simulink model "sitlpmpc"  (R2025a)
settings: Solver=FixedStepAuto  StartTime=0.0  StopTime=inf  RelTol=1e-3  EnableMultiTasking=on
PreLoadFcn:
  | SampleTime = 1e-3;
  | isUsingSimulinkMixer=true;
libraries: px4Sensorslib x2, slpidlib x2, px4Peripheralslib x1
CloseFcn:
  | clear SampleTime;
settings Model: ExtModeTrigDuration=10  Creator=The MathWorks, Inc.  LastModifiedBy=aero
settings SolverCC: AlgebraicLoopSolver=TrustRegion  PositivePriorityOrder=on  MaxZcPerStep=1.0
settings OptimizationCC: EnhancedBackFolding=on  PassReuseOutputArgsAs=Individual arguments  ZeroExternalMemoryAtStartup=off  ZeroInternalMemoryAtStartup=off  MaxStackSize=64  OptimizeBlockOrder=speed  DifferentSizesBufferReuse=on  OptimizationCustomize=off  EfficientTunableParamExpr=on
settings DebuggingCC: ParameterPrecisionLossMsg=none  ParameterTunabilityLossMsg=error  UnconnectedInputMsg=warning  UnconnectedOutputMsg=warning  UnconnectedLineMsg=warning  SubsystemReferenceDiagnosticForUnitTest=warning
settings HardwareCC: ProdBitPerPointer=32.0  ProdBitPerSizeT=32.0  ProdBitPerPtrDiffT=32.0  ProdLargestAtomicInteger=Long  ProdLargestAtomicFloat=Double  ProdWordSize=32.0  ProdLongLongMode=on  ProdHWDeviceType=ARM Compatible->ARM Cortex
settings ModelReferenceCC: EnableRefExpFcnMdlSchedulingChecks=on
settings SFSimCC: MATLABDynamicMemAlloc=off  SimTargetLang=C++  SimDLTargetLibrary=mkl-dnn
settings RTWCC: SystemTargetFile=ert.tlc  HardwareBoard=PX4 Host Target  TLCOptions="-aInlineSetEventsForThisBaseRateFcn=TLC_FALSE -aSuppressMultiTaskScheduler=TLC_FALSE  -aRateBasedStepFcn=0"  TemplateMakefile=ert_default_tmf  Toolchain=GNU Tools for PX4 Autopilots  PortableWordSizes=on  TargetLang=C++  GPUComputeCapability=3.5  DLArmComputeVersion=19.05  Description=Embedded Coder
settings CodeAppCC: ForceParamTrailComments=on  IgnoreCustomStorageClasses=off  OperatorAnnotations=on  SimulinkDataObjDesc=on  SFDataObjDesc=on  InsertBlockDesc=on
settings ERTTargetCC: ExtModeTransport=2.0  InlinedParameterPlacement=Hierarchical

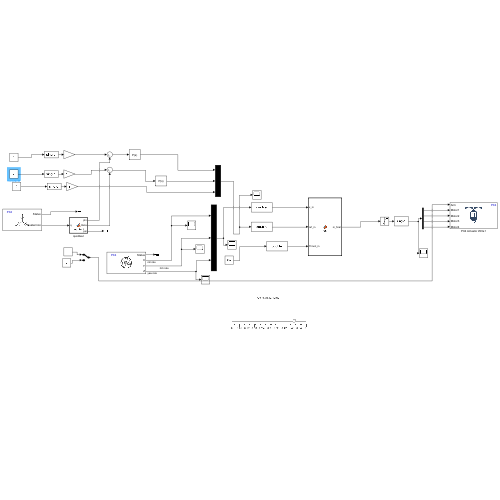
[thumbnail: Simulink's stored preview of the top-level diagram]
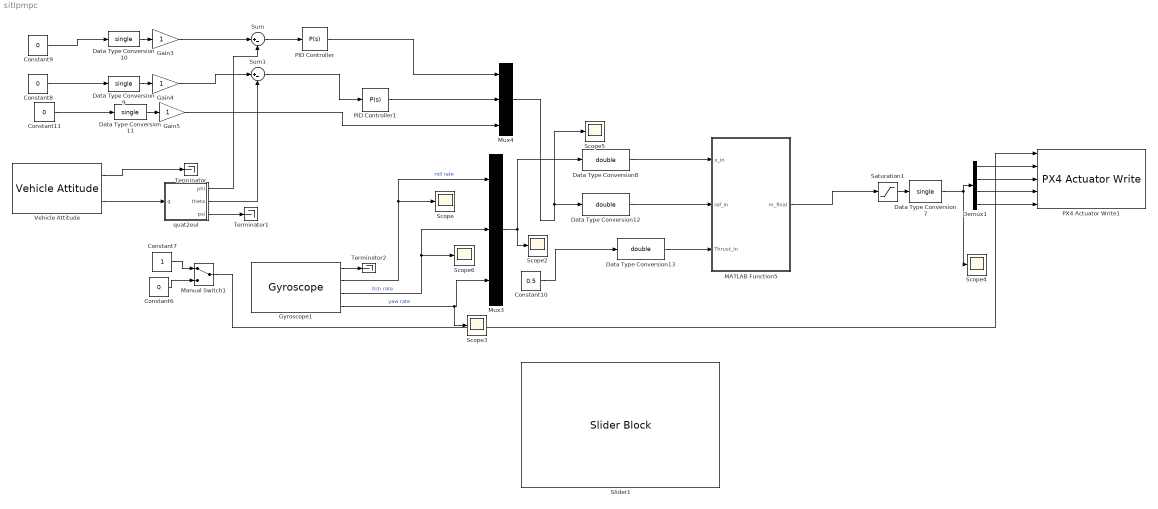
== system sitlpmpc ==
  Constant10 : Constant  Value=0.5
  Constant11 : Constant  Value=0
  Constant6 : Constant  Value=0  OutDataTypeStr=boolean
  Constant7 : Constant  OutDataTypeStr=boolean
  Constant8 : Constant  Value=0
  Constant9 : Constant  Value=0
  Data Type Conversion{7,9..11} (4 alike) : DataTypeConversion  OutDataTypeStr=single  SaturateOnIntegerOverflow=off  RndMeth=Floor
  Data Type Conversion12 : DataTypeConversion  OutDataTypeStr=double  SaturateOnIntegerOverflow=off  RndMeth=Floor  LockScale=on
  Data Type Conversion13 : DataTypeConversion  OutDataTypeStr=double  SaturateOnIntegerOverflow=off  RndMeth=Floor  LockScale=on
  Data Type Conversion8 : DataTypeConversion  OutDataTypeStr=double  SaturateOnIntegerOverflow=off  RndMeth=Floor  LockScale=on
  Demux1 : Demux
  Gain3 : Gain
  Gain4 : Gain
  Gain5 : Gain
  Gyroscope1 : px4Sensorslib/Gyroscope  uorbTimeStamp=off  BlockingMode=off  BlockTimeout=1e-3  sampleTime=0.001
  MATLAB Function5 : MATLAB Function  TreatAsAtomicUnit=on
  Manual Switch1 : ManualSwitch
  Mux3 : Mux  Inputs=3
  Mux4 : Mux  Inputs=3
  PID Controller : slpidlib/PID Controller  Controller=P  Form=Parallel  TimeDomain=Continuous-time  UseExternalTs=off  SampleTime=-1  IntegratorMethod=Forward Euler  FilterMethod=Forward Euler  ControllerParametersSource=internal  P=0.25  I=1  UseKiTs=off  D=0  UseExternalDerivativeSource=off  N=100  UseFilter=on  TunerSelectOption=Transfer Function Based (PID Tuner App)  InitialConditionSource=internal  InitialConditionForIntegrator=0  InitialConditionForFilter=0  DifferentiatorICPrevScaledInput=0  ExternalReset=none  TrackingMode=off  Kt=1  LimitOutput=off  SatLimitsSource=internal  UpperSaturationLimit=inf  LowerSaturationLimit=-inf  LinearizeAsGain=on  AntiWindupMode=none  Kb=1  LimitIntegrator=off  UpperIntegratorSaturationLimit=inf  LowerIntegratorSaturationLimit=-inf  POutMin=[]  POutMax=[]  IOutMin=[]  IOutMax=[]  DOutMin=[]  DOutMax=[]  NOutMin=[]  NOutMax=[]  SumOutMin=[]  SumOutMax=[]  SaturationOutMin=[]  SaturationOutMax=[]  PParamMin=[]  PParamMax=[]  IParamMin=[]  IParamMax=[]  DParamMin=[]  DParamMax=[]  NParamMin=[]  NParamMax=[]  KbParamMin=[]  KbParamMax=[]  KtParamMin=[]  KtParamMax=[]  KbOutMin=[]  KbOutMax=[]  KtOutMin=[]  KtOutMax=[]  IntegratorOutMin=[]  IntegratorOutMax=[]  FilterOutMin=[]  FilterOutMax=[]  SumI1OutMin=[]  SumI1OutMax=[]  SumI2OutMin=[]  SumI2OutMax=[]  SumI3OutMin=[]  SumI3OutMax=[]  SumI4OutMin=[]  SumI4OutMax=[]  SumDOutMin=[]  SumDOutMax=[]  DifferentiatorOutMin=[]  DifferentiatorOutMax=[]  FilterDiffOutCoefMin=[]  FilterDiffOutCoefMax=[]  ReciprocalOutMin=[]  ReciprocalOutMax=[]  SumDenOutMin=[]  SumDenOutMax=[]  SumNumOutMin=[]  SumNumOutMax=[]  DivideOutMin=[]  DivideOutMax=[]  UdiffTsProdOutMin=[]  UdiffTsProdOutMax=[]  NTsProdOutMin=[]  NTsProdOutMax=[]  UintegralTsProdOutMin=[]  UintegralTsProdOutMax=[]  UngainTsProdOutMin=[]  UngainTsProdOutMax=[]  ClampingZeroOutDataTypeStr=Inherit: Inherit via back propagation  ClampingZeroOutMin=[]  ClampingZeroOutMax=[]  FilterDenConstantOutDataTypeStr=Inherit: Inherit via back propagation  FilterDenConstantOutMin=[]  FilterDenConstantOutMax=[]  PCopyOutDataTypeStr=Inherit: Inherit via back propagation  PCopyOutMin=[]  PCopyOutMax=[]  NCopyOutDataTypeStr=Inherit: Inherit via back propagation  NCopyOutMin=[]  NCopyOutMax=[]  IntegratorContinuousStateAttributes=''  IntegratorStateMustResolveToSignalObject=off  IntegratorRTWStateStorageClass=Auto  FilterContinuousStateAttributes=''  FilterStateMustResolveToSignalObject=off  FilterRTWStateStorageClass=Auto  ParallelPVariant=InternalParameters  IdealPVariant=Disabled  IVariant=Disabled  DVariant=Disabled  IntegratorVariant=Disabled  SatVariant=Disabled  AWVariant=Disabled  PCopyVariant=Disabled  TRVariant=Disabled  FdbkBlocksVariant=Forward  IdealPFdbkVariant=Disabled  SatFdbkVariant=Disabled  DerivativeFilterVariant=Disabled  NVariant=Disabled  NCopyVariant=Disabled_SignalSpec  FilterICVariant=Disabled  IntegratorICVariant=Disabled  ExternalResetVariant=Disabled  TRSumVariant=Passthrough  SumFdbkVariant=Disabled  SumVariant=Passthrough_P  TsampFilterVariant=InternalTs  TsampNgainVariant=Passthrough  TsampIntegralVariant=Disabled_SignalSpec  ExternalSaturationOutDataTypeStr=Inherit: Same as second input  DerivativeSourceVariant=Disabled  PreIntVariant=InternalPreInt
  PID Controller1 : slpidlib/PID Controller  Controller=P  Form=Parallel  TimeDomain=Continuous-time  UseExternalTs=off  SampleTime=-1  IntegratorMethod=Forward Euler  FilterMethod=Forward Euler  ControllerParametersSource=internal  P=0.25  I=1  UseKiTs=off  D=0  UseExternalDerivativeSource=off  N=100  UseFilter=on  TunerSelectOption=Transfer Function Based (PID Tuner App)  InitialConditionSource=internal  InitialConditionForIntegrator=0  InitialConditionForFilter=0  DifferentiatorICPrevScaledInput=0  ExternalReset=none  TrackingMode=off  Kt=1  LimitOutput=off  SatLimitsSource=internal  UpperSaturationLimit=inf  LowerSaturationLimit=-inf  LinearizeAsGain=on  AntiWindupMode=none  Kb=1  LimitIntegrator=off  UpperIntegratorSaturationLimit=inf  LowerIntegratorSaturationLimit=-inf  POutMin=[]  POutMax=[]  IOutMin=[]  IOutMax=[]  DOutMin=[]  DOutMax=[]  NOutMin=[]  NOutMax=[]  SumOutMin=[]  SumOutMax=[]  SaturationOutMin=[]  SaturationOutMax=[]  PParamMin=[]  PParamMax=[]  IParamMin=[]  IParamMax=[]  DParamMin=[]  DParamMax=[]  NParamMin=[]  NParamMax=[]  KbParamMin=[]  KbParamMax=[]  KtParamMin=[]  KtParamMax=[]  KbOutMin=[]  KbOutMax=[]  KtOutMin=[]  KtOutMax=[]  IntegratorOutMin=[]  IntegratorOutMax=[]  FilterOutMin=[]  FilterOutMax=[]  SumI1OutMin=[]  SumI1OutMax=[]  SumI2OutMin=[]  SumI2OutMax=[]  SumI3OutMin=[]  SumI3OutMax=[]  SumI4OutMin=[]  SumI4OutMax=[]  SumDOutMin=[]  SumDOutMax=[]  DifferentiatorOutMin=[]  DifferentiatorOutMax=[]  FilterDiffOutCoefMin=[]  FilterDiffOutCoefMax=[]  ReciprocalOutMin=[]  ReciprocalOutMax=[]  SumDenOutMin=[]  SumDenOutMax=[]  SumNumOutMin=[]  SumNumOutMax=[]  DivideOutMin=[]  DivideOutMax=[]  UdiffTsProdOutMin=[]  UdiffTsProdOutMax=[]  NTsProdOutMin=[]  NTsProdOutMax=[]  UintegralTsProdOutMin=[]  UintegralTsProdOutMax=[]  UngainTsProdOutMin=[]  UngainTsProdOutMax=[]  ClampingZeroOutDataTypeStr=Inherit: Inherit via back propagation  ClampingZeroOutMin=[]  ClampingZeroOutMax=[]  FilterDenConstantOutDataTypeStr=Inherit: Inherit via back propagation  FilterDenConstantOutMin=[]  FilterDenConstantOutMax=[]  PCopyOutDataTypeStr=Inherit: Inherit via back propagation  PCopyOutMin=[]  PCopyOutMax=[]  NCopyOutDataTypeStr=Inherit: Inherit via back propagation  NCopyOutMin=[]  NCopyOutMax=[]  IntegratorContinuousStateAttributes=''  IntegratorStateMustResolveToSignalObject=off  IntegratorRTWStateStorageClass=Auto  FilterContinuousStateAttributes=''  FilterStateMustResolveToSignalObject=off  FilterRTWStateStorageClass=Auto  ParallelPVariant=InternalParameters  IdealPVariant=Disabled  IVariant=Disabled  DVariant=Disabled  IntegratorVariant=Disabled  SatVariant=Disabled  AWVariant=Disabled  PCopyVariant=Disabled  TRVariant=Disabled  FdbkBlocksVariant=Forward  IdealPFdbkVariant=Disabled  SatFdbkVariant=Disabled  DerivativeFilterVariant=Disabled  NVariant=Disabled  NCopyVariant=Disabled_SignalSpec  FilterICVariant=Disabled  IntegratorICVariant=Disabled  ExternalResetVariant=Disabled  TRSumVariant=Passthrough  SumFdbkVariant=Disabled  SumVariant=Passthrough_P  TsampFilterVariant=InternalTs  TsampNgainVariant=Passthrough  TsampIntegralVariant=Disabled_SignalSpec  ExternalSaturationOutDataTypeStr=Inherit: Same as second input  DerivativeSourceVariant=Disabled  PreIntVariant=InternalPreInt
  PX4 Actuator Write1 : px4Peripheralslib/PX4 Actuator Write  Motor1Enable=on  Motor2Enable=on  Motor3Enable=on  Motor4Enable=on  Motor5Enable=off  Motor6Enable=off  Motor7Enable=off  Motor8Enable=off  Motor9Enable=off  Motor10Enable=off  Motor11Enable=off  Motor12Enable=off  IsMotorArray=off  Servo1Enable=off  Servo2Enable=off  Servo3Enable=off  Servo4Enable=off  Servo5Enable=off  Servo6Enable=off  Servo7Enable=off  Servo8Enable=off  IsServoArray=off
  Saturation1 : Saturate  UpperLimit=1  LowerLimit=0
  Scope{,2..6} (6 alike) : Scope
      Scope settings: ActiveDisplayYMinimum=-0.048647073097527027  ActiveDisplayYMaximum=0.043675837107002735
      Scope2 settings: ActiveDisplayYMinimum=-0.62053689360618591  ActiveDisplayYMaximum=0.55083355307579041
      Scope3 settings: ActiveDisplayYMinimum=-1  ActiveDisplayYMaximum=1  DataLoggingVariableName=ScopeData3
      Scope4 settings: ActiveDisplayYMinimum=0.057510972242240666  ActiveDisplayYMaximum=0.55490137269269046  DataLoggingVariableName=ScopeData4
      Scope5 settings: ActiveDisplayYMinimum=-3.3246570702222038  ActiveDisplayYMaximum=4.6404233658291121  DataLoggingVariableName=ScopeData5
      Scope6 settings: ActiveDisplayYMinimum=-1  ActiveDisplayYMaximum=1  DataLoggingVariableName=ScopeData6
  Slider1 : SliderBlock  ScaleMax=0.6
  Sum : Sum  Inputs=|+-
  Sum1 : Sum  Inputs=|+-
  Terminator : Terminator
  Terminator1 : Terminator
  Terminator2 : Terminator
  Vehicle Attitude : px4Sensorslib/Vehicle Attitude  rollRate=off  pitchRate=off  yawRate=off  quaternion=on  uorbTimeStamp=off  BlockingMode=off  BlockTimeout=0.001  sampleTime=0.001
  quat2eul : MATLAB Function  TreatAsAtomicUnit=on
  wires:
  Data Type Conversion13/1 -> MATLAB Function5/3(Thrust_in)
  Data Type Conversion8/1 -> MATLAB Function5/1(x_in)
  Demux1/1 -> PX4 Actuator Write1/2
  Constant11/1 -> Data Type Conversion11/1
  Data Type Conversion10/1 -> Gain3/1
  Mux3/1 -> Scope2/1, Data Type Conversion8/1
  Constant8/1 -> Data Type Conversion9/1
  Data Type Conversion9/1 -> Gain4/1
  Constant9/1 -> Data Type Conversion10/1
  Constant10/1 -> Data Type Conversion13/1
  Mux4/1 -> Scope5/1, Data Type Conversion12/1
  Data Type Conversion7/1 -> Demux1/1, Scope4/1
  Demux1/4 -> PX4 Actuator Write1/5
  Saturation1/1 -> Data Type Conversion7/1
  Gyroscope1/4 -> Scope3/1, Mux3/3  "yaw rate"
  Gyroscope1/1 -> Terminator2/1
  Gyroscope1/2 -> Scope/1, Mux3/1  "roll rate"
  Constant6/1 -> Manual Switch1/2
  Data Type Conversion12/1 -> MATLAB Function5/2(ref_in)
  Constant7/1 -> Manual Switch1/1
  Demux1/3 -> PX4 Actuator Write1/4
  Data Type Conversion11/1 -> Gain5/1
  Gyroscope1/3 -> Mux3/2, Scope6/1  "itch rate"
  Demux1/2 -> PX4 Actuator Write1/3
  MATLAB Function5/1(m_final) -> Saturation1/1
  Manual Switch1/1 -> PX4 Actuator Write1/1
  Vehicle Attitude/2 -> quat2eul/1(q)
  Vehicle Attitude/1 -> Terminator/1
  Gain3/1 -> Sum/1
  Gain4/1 -> Sum1/1
  Gain5/1 -> Mux4/3
  Sum/1 -> PID Controller/1
  PID Controller/1 -> Mux4/1
  quat2eul/1(phi) -> Sum/2
  quat2eul/2(theta) -> Sum1/2
  quat2eul/3(psi) -> Terminator1/1
  Sum1/1 -> PID Controller1/1
  PID Controller1/1 -> Mux4/2

== matlab function sitlpmpc/MATLAB Function5 ==
  data: x_in input; m_final output; ref_in input; Thrust_in input
function m_final = fcn(x_in, ref_in, Thrust_in)
%#codegen

% --- CONFIGURACIÓN ESTÁTICA ---
persistent A B Phi F_f H M options lb ub Q_big
    
if isempty(A)
    % 1. Matrices del sistema
    A = [-0.935710267868369	0.114535661043099	4.926101069998020;
        -0.003429981478181	-1.040331777969572	2.779697729794189;
        -0.093493041620156	-0.275240626618720	1.498523193279717];
    B = [-1.904610791203760	-0.587512074882609	-2.268399108168063;
        -0.394955416789158	-1.757390846313468	-1.171599117715514;
        -0.076794484292644	-0.219181465035995	-0.214112941381796];

        
    % Pre-dimensionado total (N=6, nx=3, nu=3 -> 18)
    F_mat = zeros(18, 3);
    Phi_mat = zeros(18, 18);
    Q_big_mat = zeros(18, 18);
    R_big_mat = zeros(18, 18);
    
    Q_inst = eye(3) * 1; 
    R_inst = eye(3) * 2; 
        
    % Llenado de matrices con índices fijos para el compilador
    for i = 1:6
        row = (i-1)*3 + (1:3); % Esto es aceptado por Coder
        F_mat(row, :) = A^i;
        Q_big_mat(row, row) = Q_inst;
        R_big_mat(row, row) = R_inst;
        
        for j = 1:i
            col = (j-1)*3 + (1:3);
            Phi_mat(row, col) = A^(i-j) * B;
        end
    end
        
    H = 2 * (Phi_mat' * Q_big_mat * Phi_mat + R_big_mat);
    F_f = 2 * Phi_mat' * Q_big_mat * F_mat;
    Phi = Phi_mat; 
    Q_big = Q_big_mat;
        
    M = [ -1,  1,  1, -1; 
           1, -1,  1, -1; 
          -1, -1,  1,  1; 
           1,  1,  1,  1 ];
           
    options = optimoptions('quadprog', 'Algorithm', 'active-set', 'Display', 'off');
    
    % Definición directa de límites
    lb = -2 * ones(18, 1); 
    ub =  2 * ones(18, 1);
end

% --- PROCESAMIENTO ---
x = double(x_in(:));
ref_vec = double(ref_in(:));
Thrust_Cmd = double(Thrust_in);

% --- LÓGICA MPC ---
U0 = zeros(18, 1); 
Ref_seq = repmat(ref_vec, 6, 1);
f = F_f * x - (2 * Phi' * Q_big * Ref_seq);
    
[U_sol, ~, exitflag] = quadprog(H, f, [], [], [], [], lb, ub, U0, options);
    
u = zeros(3,1);
if exitflag > 0
    u = U_sol(1:3);
end
    
% Mezcla final
u_total = [u(1); u(2); u(3); Thrust_Cmd * 4]; 
m_calc = M \ u_total; 
m_final = max(min(m_calc, 1.0), 0.0);

end

== matlab function sitlpmpc/quat2eul ==
  data: q input; phi output; theta output; psi output
function [phi,theta,psi] = quat2eul(q)

% Quaternion conversion to Euler angles based on the PX4 Firmware v1.10.2
% release.

phi = atan2(2*(q(1)*q(2) + q(3)* q(4)), q(1)^2 - q(2)^2 - q(3)^2 + q(4)^2);
theta = asin(-2*(q(2)*q(4) - q(1)*q(3)));
psi = atan2(2*(q(2)*q(3) + q(1)* q(4)), q(1)^2 + q(2)^2 - q(3)^2 - q(4)^2);
end
